simulink model "sistema_completo_nl"  (R2019a)
settings: Solver=VariableStepAuto  StartTime=0.0  StopTime=10.0  RelTol=1e-3
values from neighbouring files (symbols this model uses):
  alpha_cu = 3.9e-3    (= 0.0039)    [parametros_de_sistema.m]    (also in sistema_completo_nl_script.m = 0.39)
  b_eq = b_m + b_l/r^2    (= 1.5e-05)    [parametros_de_sistema.m]    (also in sistema_completo_nl_script.m)
  C_ts = 0.818    [parametros_de_sistema.m]    (also in sistema_completo_nl_script.m)
  dT_l = 6.28    [parametros_de_sistema.m]    (also in sistema_completo_nl_script.m)
  J_eq = J_m + J_l/r^2    (= 5.65099476805e-06)    [parametros_de_sistema.m]    (also in sistema_completo_nl_script.m)
  L_d = 6.6e-3    (= 0.0066)    [parametros_de_sistema.m]    (also in sistema_completo_nl_script.m)
  L_ls = 0.8e-3    (= 0.0008)    [parametros_de_sistema.m]    (also in sistema_completo_nl_script.m)
  L_q = 5.8e-3    (= 0.0058)    [parametros_de_sistema.m]    (also in sistema_completo_nl_script.m)
  lambda_m = 0.01546    [parametros_de_sistema.m]    (also in sistema_completo_nl_script.m)
  P_p = 3    [parametros_de_sistema.m]    (also in sistema_completo_nl_script.m)
  r = 314.3008    [parametros_de_sistema.m]    (also in sistema_completo_nl_script.m)
  R_s_40 = 1.02    [parametros_de_sistema.m]    (also in sistema_completo_nl_script.m)
  R_ts_amb = 146.7    [parametros_de_sistema.m]    (also in sistema_completo_nl_script.m)
libraries: eeTransforms x1
settings Model: Creator=pedro  LastModifiedBy=pedro

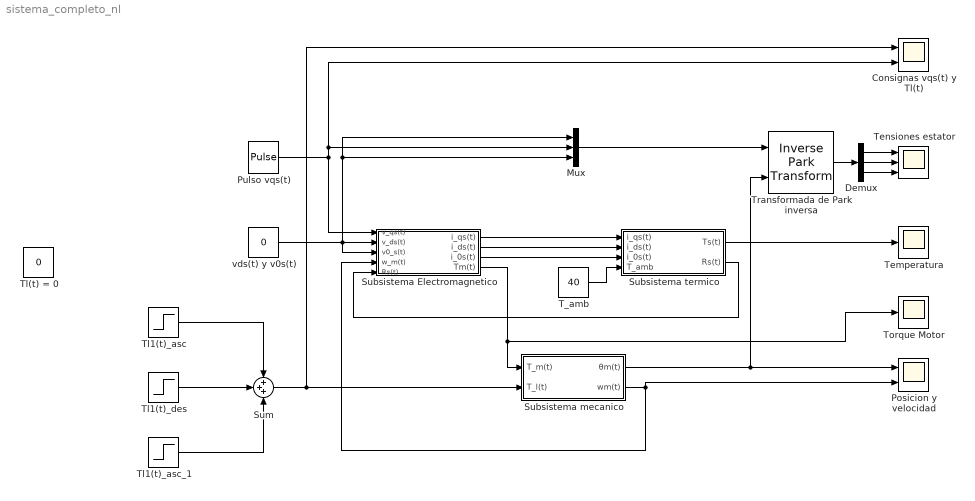
== system sistema_completo_nl ==
  Consignas vqs(t) y Tl(t) : Scope  NumInputPorts=2
  Demux : Demux  Outputs=3
  Mux : Mux  Inputs=3
  Posicion y velocidad : Scope  NumInputPorts=2
  Pulso vqs(t) : DiscretePulseGenerator  PulseType=Time based  Amplitude=19.596  Period=3  PulseWidth=20  PhaseDelay=0.1
  Subsistema Electromagnetico : Subsystem
  "Subsistema mecanico " : Subsystem
  "Subsistema termico " : Subsystem
  Sum : Sum  Inputs=+++
  T_amb : Constant  Value=40
  Temperatura : Scope
  Tensiones estator : Scope  NumInputPorts=3
  Tl(t) = 0 : Constant  Value=0
  Tl1(t)_asc : Step  Time=0  After=dT_l  SampleTime=0
  Tl1(t)_asc_1 : Step  Time=0.9  After=dT_l  SampleTime=0
  "Tl1(t)_des " : Step  Time=0.3  After=-2*dT_l  SampleTime=0
  Torque Motor : Scope
  "Transformada de Park inversa " : eeTransforms/Inverse Park Transform  AxisAlignment=Q-axis  PowerInvariant=off
      settings: SourceProductName=Simscape Electrical
  vds(t) y v0s(t) : Constant  Value=0
  wires:
  "Subsistema mecanico "/1(θm(t)) -> Posicion y velocidad/1, "Transformada de Park inversa "/2
  Subsistema Electromagnetico/4(Tm(t)) -> Torque Motor/1, "Subsistema mecanico "/1("T_m(t) ")
  Subsistema Electromagnetico/1("i_qs(t) ") -> "Subsistema termico "/1("i_qs(t) ")
  Subsistema Electromagnetico/2(i_ds(t)) -> "Subsistema termico "/2("i_ds(t) ")
  Subsistema Electromagnetico/3("i_0s(t) ") -> "Subsistema termico "/3(i_0s(t))
  "Subsistema mecanico "/2(wm(t)) -> Posicion y velocidad/2, Subsistema Electromagnetico/4(w_m(t))
  "Subsistema termico "/1(Ts(t)) -> Temperatura/1
  T_amb/1 -> "Subsistema termico "/4(T_amb)
  vds(t) y v0s(t)/1 -> Subsistema Electromagnetico/3(v0_s(t)), Mux/3, Mux/1, Subsistema Electromagnetico/2(v_ds(t))
  Pulso vqs(t)/1 -> Consignas vqs(t) y Tl(t)/2, Mux/2, Subsistema Electromagnetico/1(v_qs(t))
  Mux/1 -> "Transformada de Park inversa "/1
  "Transformada de Park inversa "/1 -> Demux/1
  Demux/1 -> Tensiones estator/1
  Demux/2 -> Tensiones estator/2
  Demux/3 -> Tensiones estator/3
  Sum/1 -> Consignas vqs(t) y Tl(t)/1, "Subsistema mecanico "/2("T_l(t) ")
  "Subsistema termico "/2(Rs(t)) -> Subsistema Electromagnetico/5("Rs(t) ")
  Tl1(t)_asc/1 -> Sum/1
  "Tl1(t)_des "/1 -> Sum/2
  Tl1(t)_asc_1/1 -> Sum/3

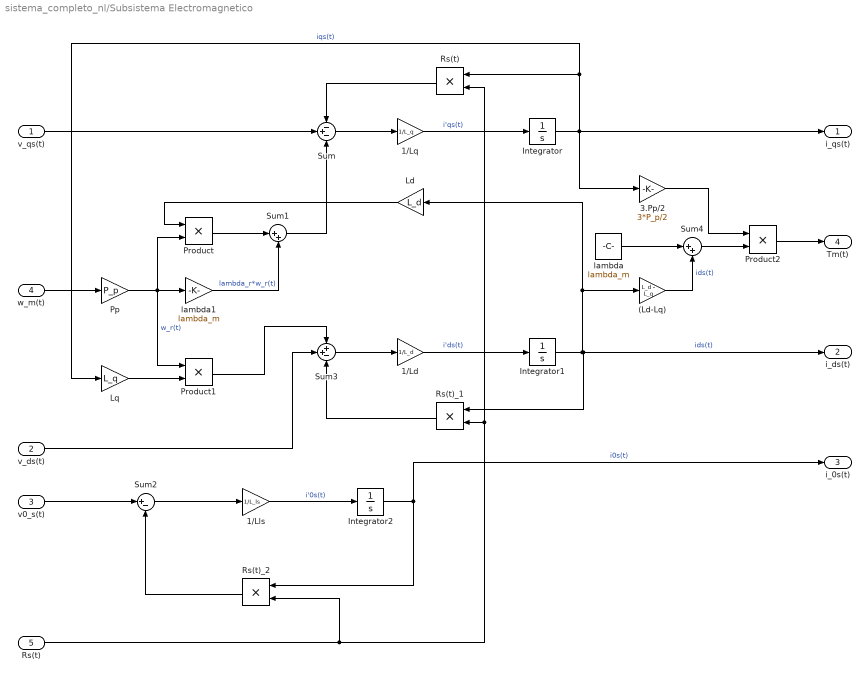
== system sistema_completo_nl/Subsistema Electromagnetico ==
  v_qs(t) : Inport
  v_ds(t) : Inport  Port=2
  v0_s(t) : Inport  Port=3
  w_m(t) : Inport  Port=4
  "Rs(t) " : Inport  Port=5
  (Ld-Lq) : Gain  Gain=L_d - L_q
  1/Ld : Gain  Gain=1/L_d
  1/Lls : Gain  Gain=1/L_ls
  1/Lq : Gain  Gain=1/L_q
  3.Pp/2 : Gain  Gain=3*P_p/2
  Integrator : Integrator
  Integrator1 : Integrator
  Integrator2 : Integrator
  Ld : Gain  Gain=L_d
  Lq : Gain  Gain=L_q
  Pp : Gain  Gain=P_p
  Product : Product
  Product1 : Product
  Product2 : Product
  Rs(t) : Product
  Rs(t)_1 : Product
  Rs(t)_2 : Product
  Sum : Sum  Inputs=-+-
  Sum1 : Sum  Inputs=|++
  Sum2 : Sum  Inputs=|+-
  Sum3 : Sum  Inputs=++-
  Sum4 : Sum  Inputs=|++
  lambda : Constant  Value=lambda_m
  lambda1 : Gain  Gain=lambda_m
  "i_qs(t) " : Outport
  i_ds(t) : Outport  Port=2
  "i_0s(t) " : Outport  Port=3
  Tm(t) : Outport  Port=4
  wires:
  w_m(t)/1 -> Pp/1
  Pp/1 -> Product1/1, Product/2, lambda1/1  "w_r(t)"
  Sum/1 -> 1/Lq/1
  1/Lq/1 -> Integrator/1  "i'qs(t)"
  Sum1/1 -> Sum/3
  v_qs(t)/1 -> Sum/2
  Integrator/1 -> Lq/1, Rs(t)/1, 3.Pp/2/1, "i_qs(t) "/1  "iqs(t)"
  lambda1/1 -> Sum1/2  "lambda_r*w_r(t)"
  Product/1 -> Sum1/1
  v_ds(t)/1 -> Sum3/2
  Sum3/1 -> 1/Ld/1
  Product1/1 -> Sum3/1
  1/Ld/1 -> Integrator1/1  "i'ds(t)"
  Integrator1/1 -> Ld/1, (Ld-Lq)/1, Rs(t)_1/1, i_ds(t)/1  "ids(t)"
  Lq/1 -> Product1/2
  Ld/1 -> Product/1
  v0_s(t)/1 -> Sum2/1
  Rs(t)_2/1 -> Sum2/2
  Sum2/1 -> 1/Lls/1
  1/Lls/1 -> Integrator2/1  "i'0s(t)"
  Integrator2/1 -> Rs(t)_2/1, "i_0s(t) "/1  "i0s(t)"
  (Ld-Lq)/1 -> Sum4/2  "ids(t)"
  lambda/1 -> Sum4/1
  Sum4/1 -> Product2/2
  Product2/1 -> Tm(t)/1
  3.Pp/2/1 -> Product2/1
  "Rs(t) "/1 -> Rs(t)_2/2, Rs(t)/2, Rs(t)_1/2
  Rs(t)_1/1 -> Sum3/3
  Rs(t)/1 -> Sum/1

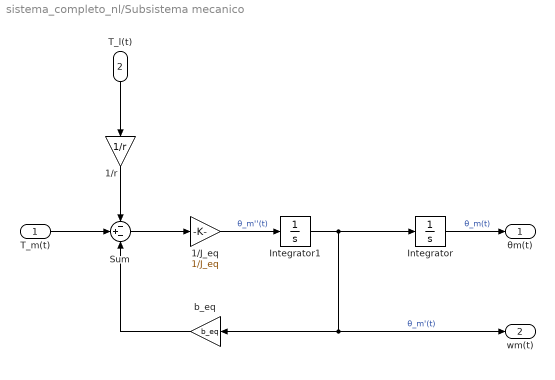
== system sistema_completo_nl/Subsistema mecanico  ==
  "T_m(t) " : Inport
  "T_l(t) " : Inport  Port=2
  "1/J_eq " : Gain  Gain=1/J_eq
  1/r : Gain  Gain=1/r
  Integrator : Integrator
  Integrator1 : Integrator
  Sum : Sum  Inputs=-+-
  b_eq : Gain  Gain=b_eq
  θm(t) : Outport
  wm(t) : Outport  Port=2
  wires:
  Integrator1/1 -> b_eq/1, wm(t)/1, Integrator/1  "θ_m'(t)"
  Sum/1 -> "1/J_eq "/1
  b_eq/1 -> Sum/3
  "1/J_eq "/1 -> Integrator1/1  "θ_m''(t)"
  Integrator/1 -> θm(t)/1  "θ_m(t)"
  "T_m(t) "/1 -> Sum/2
  "T_l(t) "/1 -> 1/r/1
  1/r/1 -> Sum/1

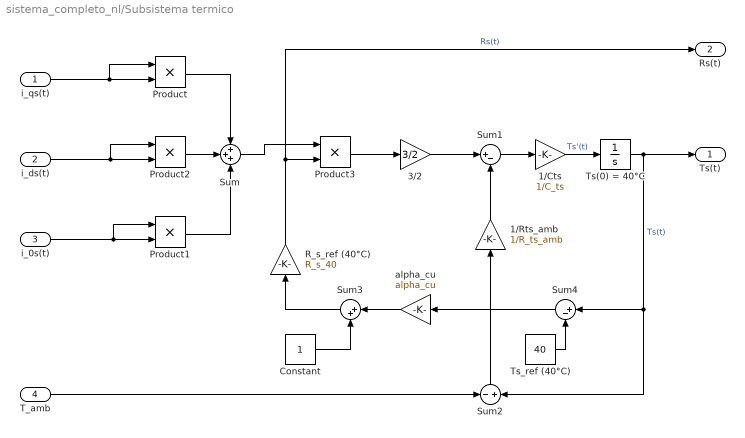
== system sistema_completo_nl/Subsistema termico  ==
  "i_qs(t) " : Inport
  "i_ds(t) " : Inport  Port=2
  i_0s(t) : Inport  Port=3
  T_amb : Inport  Port=4
  1/Cts : Gain  Gain=1/C_ts
  1/Rts_amb : Gain  Gain=1/R_ts_amb
  3/2 : Gain  Gain=3/2
  Constant : Constant
  Product{,1..3} (4 alike) : Product
  R_s_ref (40°C) : Gain  Gain=R_s_40
  Sum : Sum  Inputs=+++
  Sum1 : Sum  Inputs=|+-
  Sum2 : Sum  Inputs=-|+
  Sum3 : Sum  Inputs=|++
  Sum4 : Sum  Inputs=|+-
  Ts(0) = 40°C : Integrator  InitialCondition=40
  Ts_ref (40°C) : Constant  Value=40
  alpha_cu : Gain  Gain=alpha_cu
  Ts(t) : Outport
  Rs(t) : Outport  Port=2
  wires:
  i_0s(t)/1 -> Product1/1, Product1/2
  "i_ds(t) "/1 -> Product2/1, Product2/2
  "i_qs(t) "/1 -> Product/1, Product/2
  Product/1 -> Sum/1
  Product2/1 -> Sum/2
  Product1/1 -> Sum/3
  Ts(0) = 40°C/1 -> Sum4/1, Sum2/2, Ts(t)/1  "Ts(t)"
  T_amb/1 -> Sum2/1
  Sum2/1 -> 1/Rts_amb/1
  1/Rts_amb/1 -> Sum1/2
  Sum1/1 -> 1/Cts/1
  1/Cts/1 -> Ts(0) = 40°C/1  "Ts'(t)"
  Constant/1 -> Sum3/2
  alpha_cu/1 -> Sum3/1
  Sum3/1 -> R_s_ref (40°C)/1
  R_s_ref (40°C)/1 -> Rs(t)/1, Product3/2  "Rs(t)"
  Sum/1 -> Product3/1
  Product3/1 -> 3/2/1
  3/2/1 -> Sum1/1
  Ts_ref (40°C)/1 -> Sum4/2
  Sum4/1 -> alpha_cu/1
